simulink model "ChiefMaster_TTC580"  (R2022b)
settings: Solver=FixedStepAuto  StartTime=0.0  StopTime=10  FixedStep=0.01  RelTol=1e-3
values from neighbouring files (symbols this model uses):
  BattBox1_No = single(1)    [Parameters.m]
  BattBox2_No = single(2)    [Parameters.m]
  BattBox3_No = single(3)    [Parameters.m]
  CurrentLB = single(-3)    [Parameters.m]
  CurrentReductionConstant_Lvl0 = single(0.03)    [Parameters.m]
  CurrentReductionConstant_Lvl1 = single(0.05)    [Parameters.m]
  CurrentReductionConstant_Lvl2 = single(0.07)    [Parameters.m]
  CurrentReductionConstant_Lvl3 = single(0.1)    [Parameters.m]
  CurrentUB = single(3)    [Parameters.m]
  DCHV_Minus_In_Delay_ms = single(500)    [Parameters.m]
  FL_sHVC_CellBalanceVoltage_mV = single(3500)    [Parameters.m]
  FL_sInrushCurrent_dividebyzero = single(0.00001)    [Parameters.m]
  FL_u8HMI_BuzzerTimer = uint8(3)    [Parameters.m]
  IP_boActValue = true    [Parameters.m]
  IP_boDeactValue = false    [Parameters.m]
  IP_boInitValue = false    [Parameters.m]
  IP_s_LB = 18000    [Parameters.m]
  IP_s_UB = 22000    [Parameters.m]
  IP_sBatt1_ChargeCurrentMax_Factor = single(0.1)    [Parameters.m]
  IP_sBatt1_ChargeCurrentMax_LB = single(0)    [Parameters.m]
  IP_sBatt1_ChargeCurrentMax_Offset = single(0)    [Parameters.m]
  IP_sBatt1_ChargeCurrentMax_UB = single(6553.5)    [Parameters.m]
  IP_sBatt1_Current_Factor = single(0.1)    [Parameters.m]
  IP_sBatt1_Current_LB = single(-3276.8)    [Parameters.m]
  IP_sBatt1_Current_Offset = single(0)    [Parameters.m]
  IP_sBatt1_Current_UB = single(3276.8)    [Parameters.m]
  IP_sBatt1_DisChargeCurrentMax_Factor = single(0.1)    [Parameters.m]
  IP_sBatt1_DisChargeCurrentMax_LB = single(0)    [Parameters.m]
  IP_sBatt1_DisChargeCurrentMax_Offset = single(0)    [Parameters.m]
  IP_sBatt1_DisChargeCurrentMax_UB = single(6553.5)    [Parameters.m]
  IP_sBatt1_InsulationResistance_Factor = single(5)    [Parameters.m]
  IP_sBatt1_InsulationResistance_LB = single(0)    [Parameters.m]
  IP_sBatt1_InsulationResistance_Offset = single(0)    [Parameters.m]
  IP_sBatt1_InsulationResistance_UB = single(0)    [Parameters.m]
  IP_sBatt1_LiBa_IntResist_mOhm = single(25)    [Parameters.m]
  IP_sBatt1_SOC_Factor = single(1)    [Parameters.m]
  IP_sBatt1_SOC_LB = single(0)    [Parameters.m]
  IP_sBatt1_SOC_Offset = single(0)    [Parameters.m]
  IP_sBatt1_SOC_UB = single(100)    [Parameters.m]
  IP_sBatt1_SOH_Factor = single(1)    [Parameters.m]
  IP_sBatt1_SOH_LB = single(0)    [Parameters.m]
  IP_sBatt1_SOH_Offset = single(0)    [Parameters.m]
  IP_sBatt1_SOH_UB = single(100)    [Parameters.m]
  IP_sBatt1_Ubatt_Factor = single(0.1)    [Parameters.m]
  IP_sBatt1_Ubatt_LB = single(0)    [Parameters.m]
  IP_sBatt1_Ubatt_Offset = single(0)    [Parameters.m]
  IP_sBatt1_Ubatt_UB = single(6553.5)    [Parameters.m]
  IP_sBatt1_UserRi_Factor = single(1)    [Parameters.m]
  IP_sBatt1_UserRi_LB = single(0)    [Parameters.m]
  IP_sBatt1_UserRi_Offset = single(0)    [Parameters.m]
  IP_sBatt1_UserRi_UB = single(255)    [Parameters.m]
  IP_sBatt1_VoltageAtSensor_Factor = single(0.02)    [Parameters.m]
  IP_sBatt1_VoltageAtSensor_LB = single(0)    [Parameters.m]
  IP_sBatt1_VoltageAtSensor_Offset = single(0)    [Parameters.m]
  IP_sBatt1_VoltageAtSensor_UB = single(1310.7)    [Parameters.m]
  IP_sBatt2_LiBa_IntResist_mOhm = single(25)    [Parameters.m]
  IP_sBatt3_LiBa_IntResist_mOhm = single(25)    [Parameters.m]
  IP_sEM_LB = 2000    [Parameters.m]
  IP_sEM_UB = 8000    [Parameters.m]
  IP_sFB_LB = 5000    [Parameters.m]
  IP_sFB_UB = 10000    [Parameters.m]
  IP_sHVIL_LB = 12000    [Parameters.m]
  IP_sHVIL_UB = 15000    [Parameters.m]
  IP_sLoad_Voltage_Factor = single(1)    [Parameters.m]
  IP_sLoad_Voltage_LB = single(0)    [Parameters.m]
  IP_sLoad_Voltage_Offset = single(0)    [Parameters.m]
  IP_sLoad_Voltage_UB = single(65535)    [Parameters.m]
  IP_u8HVIL_Delay_ms = uint8(100)    [Parameters.m]
  IP_u8HW_IN_delay_ms = uint8(100)    [Parameters.m]
  IT_sInsulationSafeValue_kOhm = single(650)    [Parameters.m]
  IT_u8IMD_DelayTime_s = uint8(20)    [Parameters.m]
  MainHV_Minus_In_Delay = single(5)    [Parameters.m]
  MainHV_StatusDelay = single(5)    [Parameters.m]
  NotAvailable_uint16 = single(65535)    [Parameters.m]
  NotAvailable_uint8 = uint8(255)    [Parameters.m]
  OP_boHVIL_Supply = boolean(1)    [Parameters.m]
  SafeCurrentToCloseHV_A = single(5)    [Parameters.m]
  SafeVoltageToCloseHV_V = single(0.5)    [Parameters.m]
  UnexpectedBattChargingFcn_Available = boolean(1)    [Parameters.m]
  Voltage_NA_UB = uint16(65535)    [Parameters.m]
  VoltageSensorAvailableBB1 = boolean(0)    [Parameters.m]
  VoltageSensorAvailableBB2 = boolean(0)    [Parameters.m]
  VoltageSensorAvailableBB3 = boolean(0)    [Parameters.m]
libraries: simulink x184, Library_DataProcessing_v1_1 x167, Library_DataProcessing_v1 x142, libCM x28
(part 3 of 19)

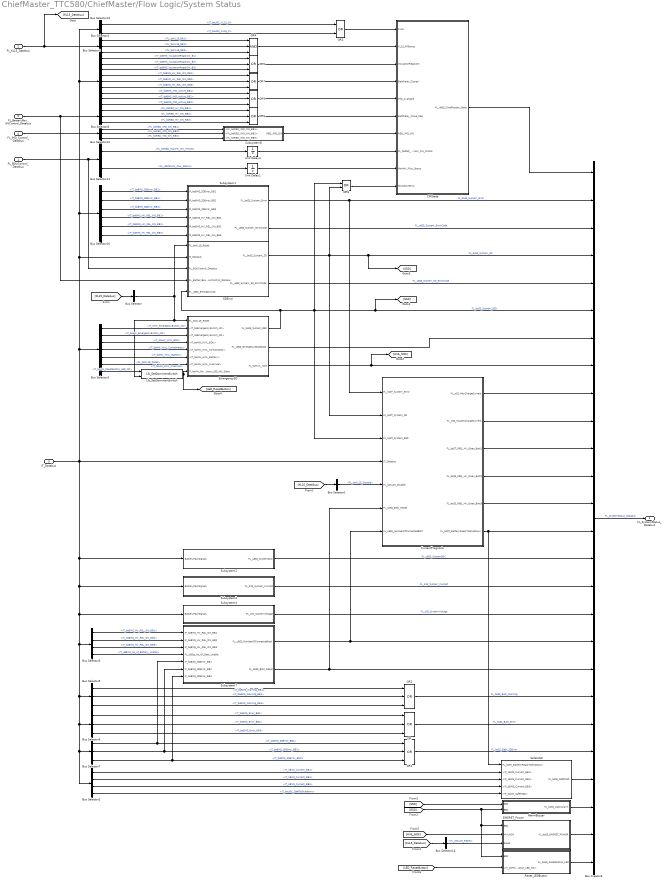
== system ChiefMaster_TTC580/ChiefMaster/Flow Logic/System Status ==
  FL_BDUControl_Databus : Inport
  FL_KL15_Databus : Inport  Port=2
  IT_Databus : Inport  Port=3
  FL_IMD_Control_Databus : Inport  Port=4
  FL_BatteryBox_HVControl_Databus : Inport  Port=5
  AlarmBuzzer : Subsystem
  Bus Creator6 : BusCreator  Inputs=26
  Bus Selector : BusSelector  OutputSignals=FL_boKL15_Reset
  Bus Selector1 : BusSelector  OutputSignals=FL_boKL15_Disable
  Bus Selector10 : BusSelector  OutputSignals=IT_BatterySignal_Databus.IT_boBMS_SDError_BB1,IT_BatterySignal_Databus.IT_boBMS_SDError_BB2,IT_BatterySignal_Databus.IT_boBMS_SDError_BB3,IT_BatterySignal_Databus.IT_boBMS_HV_REL_ON_BB1,IT_BatterySignal_Databus.IT_boBMS_HV_REL_ON_BB2,IT_BatterySignal_Databus.IT_boBMS_HV_REL_ON_BB3
  Bus Selector11 : BusSelector  OutputSignals=FL_boREQ_MainHV_ON_MINUS,FL_u8MainHV_Plus_Status
  Bus Selector12 : BusSelector  OutputSignals=FL_boREQ_IMD_ON_BB1,FL_boREQ_IMD_ON_BB2,FL_boREQ_IMD_ON_BB3
  Bus Selector13 : BusSelector  OutputSignals=IT_UDC_Databus.IT_boUDC_KL15_D,IT_UDC_Databus.IT_boUDC_KL15_C
  Bus Selector14 : BusSelector  OutputSignals=FL_boKL15_Reset
  Bus Selector2 : BusSelector  OutputSignals=IT_BatterySignal_Databus.IT_sBMS_Current_BB1,IT_BatterySignal_Databus.IT_sBMS_Current_BB2,IT_BatterySignal_Databus.IT_sBMS_Current_BB3,IT_UDC_Databus.IT_boUDC_SafeToShutdown
  Bus Selector3 : BusSelector  OutputSignals=IT_HW_Input_Databus.IT_sHW_EmergencyButton_NC,IT_HW_Input_Databus.IT_boHW_EmergencyButton_NO,IT_HW_Input_Databus.IT_boHW_HVIL_BDU,IT_HW_Input_Databus.IT_boHW_HVIL_Components,IT_HW_Input_Databus.IT_boHW_HVIL_Battery,IT_HW_Input_Databus.IT_boHW_HVIL_Overrule,IT_HW_Input_Databus.IT_boHW_ResetButton_LED_NO
  "Bus Selector3 " : BusSelector  OutputSignals=IT_BatterySignal_Databus.IT_boBMS_HV_REL_ON_BB1,IT_BatterySignal_Databus.IT_boBMS_HV_REL_ON_BB2,IT_BatterySignal_Databus.IT_boBMS_HV_REL_ON_BB3,IT_BatterySignal_Databus.IT_u8BMS_No_of_Battery_Usable
  Bus Selector4 : BusSelector  OutputSignals=FL_boKL15_BB1,FL_boKL15_BB2,FL_boKL15_BB3
  Bus Selector5 : BusSelector  OutputSignals=IT_BatterySignal_Databus.IT_boBMS_Warning_BB1,IT_BatterySignal_Databus.IT_boBMS_Warning_BB2,IT_BatterySignal_Databus.IT_boBMS_Warning_BB3
  Bus Selector6 : BusSelector  OutputSignals=IT_BatterySignal_Databus.IT_boBMS_Error_BB1,IT_BatterySignal_Databus.IT_boBMS_Error_BB2,IT_BatterySignal_Databus.IT_boBMS_Error_BB3
  Bus Selector7 : BusSelector  OutputSignals=IT_BatterySignal_Databus.IT_boBMS_SDError_BB1,IT_BatterySignal_Databus.IT_boBMS_SDError_BB2,IT_BatterySignal_Databus.IT_boBMS_SDError_BB3
  Bus Selector8 : BusSelector  OutputSignals=FL_boREQ_HV_ON_BB1,FL_boREQ_HV_ON_BB2,FL_boREQ_HV_ON_BB3
  Bus Selector9 : BusSelector  OutputSignals=IT_BatterySignal_Databus.IT_boBMS_InsulationReadyOK_B1,IT_BatterySignal_Databus.IT_boBMS_InsulationReadyOK_B2,IT_BatterySignal_Databus.IT_boBMS_InsulationReadyOK_B3,IT_BatterySignal_Databus.IT_boBMS_HV_REL_ON_BB1,IT_BatterySignal_Databus.IT_boBMS_HV_REL_ON_BB2,IT_BatterySignal_Databus.IT_boBMS_HV_REL_ON_BB3,IT_BatterySignal_Databus.IT_boBMS_IMD_Active_BB1,IT_BatterySignal_Databus.IT_boBMS_IMD_Active_BB2,IT_BatterySignal_Databus.IT_boBMS_IMD_Active_BB3
  CMState : Subsystem  TreatAsAtomicUnit=on
      settings: RTWFcnNameOpts=Use subsystem name  RTWFileNameOpts=Use subsystem name
  CurrentPrognosis : Subsystem
  EMSRET_Power : Subsystem  TreatAsAtomicUnit=on
      settings: RTWFcnNameOpts=Use subsystem name  RTWFileNameOpts=Use subsystem name
  EmergencySD : Subsystem  TreatAsAtomicUnit=on
      settings: RTWFcnNameOpts=Use subsystem name  RTWFileNameOpts=Use subsystem name
  Lib_SetDominantSwitch : Library_DataProcessing_v1_1/Lib_SetDominantSwitch  SystemSampleTime=-1  VariantActivationTime=update diagram  Latency=0  AutoFrameSizeCalculation=off
  OR{,1..2,5..7,9} (7 alike) : Logic  Operator=OR  Inputs=3  AllPortsSameDT=off  OutDataTypeStr=boolean
  OR3 : Logic  Operator=OR  AllPortsSameDT=off  OutDataTypeStr=boolean
  OR4 : Logic  Inputs=3  AllPortsSameDT=off  OutDataTypeStr=boolean
  OR8 : Logic  Operator=OR  AllPortsSameDT=off  OutDataTypeStr=boolean
  Reset_LEDButton : Subsystem
  SDError : Subsystem  TreatAsAtomicUnit=on
      settings: RTWFcnNameOpts=Use subsystem name  RTWFileNameOpts=Use subsystem name
  SafetoSD : Subsystem
  Subsystem1 : Subsystem
  Subsystem2 : Subsystem
  Subsystem3 : Subsystem
  Subsystem4 : Subsystem
  Subsystem7 : Subsystem
  Subsystem8 : Subsystem
  Unit Delay1 : UnitDelay  SampleTime=-1  HasFrameUpgradeWarning=on
  Unit Delay4 : UnitDelay  SampleTime=-1  HasFrameUpgradeWarning=on
  FL_SystemStatus_Databus : Outport
  wires:
  "Bus Selector3 "/4 -> Subsystem7/4(FL_u8Sig_No_Of_Batt_Usable)  "<IT_u8BMS_No_of_Battery_Usable>"
  Subsystem1/2(FL_u8SS_System_ErrorCode) -> Bus Creator6/3  "FL_u8SS_System_ErrorCode"
  Bus Selector10/4 -> Subsystem1/4(IP_boBMS_HV_REL_ON_BB1)  "<IT_boBMS_HV_REL_ON_BB1>"
  Subsystem7/1(FL_u8SS_NumberOfConnectedBatt) -> CurrentPrognosis/7(FL_u8SS_NumberOfConnectedBatt), Bus Creator6/18
  Bus Selector10/6 -> Subsystem1/6(IP_boBMS_HV_REL_ON_BB3)  "<IT_boBMS_HV_REL_ON_BB3>"
  Bus Selector5/1 -> OR2/1  "<IT_boBMS_Warning_BB1>"
  Subsystem1/1(FL_boSS_System_Error) -> CurrentPrognosis/1(FL_boST_System_Error), Bus Creator6/2  "FL_boSS_System_Error"
  "Bus Selector3 "/2 -> Subsystem7/2(IP_boBMS_HV_REL_ON_BB2)  "<IT_boBMS_HV_REL_ON_BB2>"
  SDError/2(FL_u8SS_System_SD_ErrorCode) -> Bus Creator6/5  "FL_u8SS_System_SD_ErrorCode"
  "Bus Selector3 "/1 -> Subsystem7/1(IP_boBMS_HV_REL_ON_BB1)  "<IT_boBMS_HV_REL_ON_BB1>"
  Bus Selector10/5 -> Subsystem1/5(IP_boBMS_HV_REL_ON_BB2)  "<IT_boBMS_HV_REL_ON_BB2>"
  Bus Selector10/1 -> Subsystem1/1(IP_boBMS_SDError_BB1)  "<IT_boBMS_SDError_BB1>"
  Bus Selector7/1 -> OR1/1, Subsystem7/5(IP_boBMS_SDError_BB1)  "<IT_boBMS_SDError_BB1>"
  "Bus Selector3 "/3 -> Subsystem7/3(IP_boBMS_HV_REL_ON_BB3)  "<IT_boBMS_HV_REL_ON_BB3>"
  Bus Selector5/2 -> OR2/2  "<IT_boBMS_Warning_BB2>"
  Bus Selector6/3 -> OR/3  "<IT_boBMS_Error_BB3>"
  Bus Selector7/3 -> Subsystem7/7(IP_boBMS_SDError_BB3), OR1/3  "<IT_boBMS_SDError_BB3>"
  Subsystem7/2(FL_boSS_BDU_Reset) -> CurrentPrognosis/6(FL_boSS_BDU_Reset), Bus Creator6/19
  Bus Selector6/2 -> OR/2  "<IT_boBMS_Error_BB2>"
  Bus Selector10/3 -> Subsystem1/3(IP_boBMS_SDError_BB3)  "<IT_boBMS_SDError_BB3>"
  OR2/1 -> Bus Creator6/20  "FL_boSS_Batt_Warning"
  OR1/1 -> Bus Creator6/22  "FL_boSS_Batt_SDError"
  Bus Selector10/2 -> Subsystem1/2(IP_boBMS_SDError_BB2)  "<IT_boBMS_SDError_BB2>"
  Bus Selector5/3 -> OR2/3  "<IT_boBMS_Warning_BB3>"
  Bus Selector6/1 -> OR/1  "<IT_boBMS_Error_BB1>"
  OR/1 -> Bus Creator6/21  "FL_boSS_Batt_Error"
  Subsystem4/1(FL_sST_SystemVoltage) -> Bus Creator6/17  "FL_sSS_SystemVoltage"
  Bus Creator6/1 -> FL_SystemStatus_Databus/1  "FL_SystemStatus_Databus"
  Bus Selector/1 -> Lib_SetDominantSwitch/2, EmergencySD/1(FL_boKL15_Reset), SDError/1(FL_boKL15_Reset)  "<FL_boKL15_Reset>"
  FL_BatteryBox_HVControl_Databus/1 -> SDError/4(FL_BatteryBox_HVControl_Databus), Bus Selector8/1
  Subsystem3/1(FL_sSS_System_Current) -> Bus Creator6/16  "FL_sSS_System_Current"
  Subsystem2/1(FL_u8SS_SystemSOC) -> Bus Creator6/15  "FL_u8SS_SystemSOC"
  CurrentPrognosis/1(FL_sSS_MaxChargeCurrent) -> Bus Creator6/9
  EmergencySD/1(FL_boSS_System_ESD) -> SDError/5(FL_u8SS_EmergencySD), CurrentPrognosis/3(FL_boST_System_ESD), OR8/1, [ESD], Bus Creator6/6  "FL_boSS_System_ESD"
  Bus Selector3/1 -> EmergencySD/2(<IT_boEmergencySwitch_NC>)  "<IT_sHW_EmergencyButton_NC>"
  SDError/1(FL_boSS_System_SD) -> OR8/2, [SSD], Bus Creator6/4, CurrentPrognosis/2(FL_boST_System_SD)  "FL_boSS_System_SD"
  Bus Selector7/2 -> Subsystem7/6(IP_boBMS_SDError_BB2), OR1/2  "<IT_boBMS_SDError_BB2>"
  CurrentPrognosis/2(FL_sSS_MaxDisChargeCurrent) -> Bus Creator6/10
  OR9/1 -> CMState/5(IMD_Available)
  Bus Selector9/9 -> OR9/3  "<IT_boBMS_IMD_Active_BB3>"
  Bus Selector9/8 -> OR9/2  "<IT_boBMS_IMD_Active_BB2>"
  Bus Selector9/7 -> OR9/1  "<IT_boBMS_IMD_Active_BB1>"
  Subsystem8/1(REQ_IMD_ON) -> CMState/7(REQ_IMD_ON)
  OR6/1 -> CMState/6(BattRelay_Close_Req)
  OR7/1 -> CMState/4(BattRelay_Closed)
  OR5/1 -> CMState/3(InsulationReadyOK)
  Unit Delay1/1 -> CMState/9(MainHV_Plus_Status)
  Bus Selector12/3 -> Subsystem8/3(<FL_boREQ_IMD_ON_BB3>)  "<FL_boREQ_IMD_ON_BB3>"
  Bus Selector12/2 -> Subsystem8/2(<FL_boREQ_IMD_ON_BB2>)  "<FL_boREQ_IMD_ON_BB2>"
  Bus Selector12/1 -> Subsystem8/1(<FL_boREQ_IMD_ON_BB1>)  "<FL_boREQ_IMD_ON_BB1>"
  OR4/1 -> CMState/2(KL15_AllBoxes)
  Unit Delay4/1 -> CMState/8(FL_boREQ_MainHV_ON_MINUS)
  OR8/1 -> CMState/10(ShutdownError)
  Bus Selector9/6 -> OR7/3  "<IT_boBMS_HV_REL_ON_BB3>"
  Bus Selector9/5 -> OR7/2  "<IT_boBMS_HV_REL_ON_BB2>"
  Bus Selector9/4 -> OR7/1  "<IT_boBMS_HV_REL_ON_BB1>"
  Bus Selector11/2 -> Unit Delay1/1  "<FL_u8MainHV_Plus_Status>"
  Bus Selector11/1 -> Unit Delay4/1  "<FL_boREQ_MainHV_ON_MINUS>"
  FL_BDUControl_Databus/1 -> Bus Selector11/1, SDError/3(FL_BDUControl_Databus)
  Bus Selector8/3 -> OR6/3  "<FL_boREQ_HV_ON_BB3>"
  Bus Selector8/2 -> OR6/2  "<FL_boREQ_HV_ON_BB2>"
  Bus Selector8/1 -> OR6/1  "<FL_boREQ_HV_ON_BB1>"
  Bus Selector9/3 -> OR5/3  "<IT_boBMS_InsulationReadyOK_B3>"
  Bus Selector9/2 -> OR5/2  "<IT_boBMS_InsulationReadyOK_B2>"
  Bus Selector9/1 -> OR5/1  "<IT_boBMS_InsulationReadyOK_B1>"
  IT_Databus/1 -> SDError/2(IT_Databus), Bus Selector13/1, Bus Selector9/1, Bus Selector10/1, Bus Selector3/1, Subsystem4/1(BatteryPackSignals), Bus Selector2/1, Bus Selector7/1, Bus Selector6/1, Bus Selector5/1, "Bus Selector3 "/1, Subsystem3/1(BatteryPackSignals), Subsystem2/1(BatteryPackSignals), CurrentPrognosis/4(IT_Databus)
  Bus Selector4/3 -> OR4/3  "<FL_boKL15_BB3>"
  Bus Selector4/2 -> OR4/2  "<FL_boKL15_BB2>"
  Bus Selector4/1 -> OR4/1  "<FL_boKL15_BB1>"
  FL_KL15_Databus/1 -> [KL15_Databus], Bus Selector4/1
  FL_IMD_Control_Databus/1 -> Bus Selector12/1
  CMState/1(FL_u8SS_ChiefMaster_State) -> Bus Creator6/1
  Bus Selector13/1 -> OR3/1  "<IT_boUDC_KL15_D>"
  Bus Selector3/2 -> EmergencySD/3(<IT_boEmergencySwitch_NO>)  "<IT_boHW_EmergencyButton_NO>"
  EmergencySD/2(FL_u8SS_EmergencyStopState) -> Bus Creator6/7
  [KL15_Databus] -> Bus Selector/1
  Bus Selector1/1 -> CurrentPrognosis/5(FL_boKL15_Disable)  "<FL_boKL15_Disable>"
  [KL15_Databus] -> Bus Selector1/1
  CurrentPrognosis/3(FL_boST_REQ_HV_Open_Batt1) -> Bus Creator6/11
  CurrentPrognosis/4(FL_boSS_REQ_HV_Open_Batt2) -> Bus Creator6/12
  CurrentPrognosis/5(FL_boSS_REQ_HV_Open_Batt3) -> Bus Creator6/13
  CurrentPrognosis/6(FL_boST_BatteryReadyToShutDown) -> Bus Creator6/14, SafetoSD/1(FL_boST_BatteryReadyToShutDown)
  SafetoSD/1(FL_boSS_SafeToSD) -> Bus Creator6/23
  Bus Selector2/1 -> SafetoSD/2(<IP_sBMS_Current_BB1>)  "<IT_sBMS_Current_BB1>"
  Bus Selector2/2 -> SafetoSD/3(<IP_sBMS_Current_BB2>)  "<IT_sBMS_Current_BB2>"
  Bus Selector2/3 -> SafetoSD/4(<IP_sBMS_Current_BB3>)  "<IT_sBMS_Current_BB3>"
  Bus Selector2/4 -> SafetoSD/5(<IP_boCM_SafeToSD>)  "<IT_boUDC_SafeToShutdown>"
  Bus Selector3/3 -> EmergencySD/4(<IT_boHW_HVIL_BDU>)  "<IT_boHW_HVIL_BDU>"
  Bus Selector3/4 -> EmergencySD/5(<IT_boHW_HVIL_Components>)  "<IT_boHW_HVIL_Components>"
  Bus Selector3/5 -> EmergencySD/6(<IT_boHW_HVIL_Battery>)  "<IT_boHW_HVIL_Battery>"
  Bus Selector3/6 -> EmergencySD/7(<IT_boHW_HVIL_Overrule>)  "<IT_boHW_HVIL_Overrule>"
  EmergencySD/3(FL_boHVIL_NOK) -> [HVIL_NOK], Bus Creator6/8
  [ESD] -> Reset_LEDButton/1(ESD), EMSRET_Power/1(ESD), AlarmBuzzer/2(ESD)
  EMSRET_Power/1(FL_boSS_EMSRET_POWER) -> Bus Creator6/25
  AlarmBuzzer/1(FL_boSS_CabinAlarm) -> Bus Creator6/24
  [HVIL_NOK] -> EMSRET_Power/2(HVILNOK)
  [SSD] -> AlarmBuzzer/1(SSD)
  Bus Selector14/1 -> EMSRET_Power/3(Reset)  "<FL_boKL15_Reset>"
  [KL15_Databus] -> Bus Selector14/1
  Bus Selector13/2 -> OR3/2  "<IT_boUDC_KL15_C>"
  OR3/1 -> CMState/1(KL15)
  Bus Selector3/7 -> Lib_SetDominantSwitch/1  "<IT_boHW_ResetButton_LED_NO>"
  Reset_LEDButton/1(FL_boSS_ResetButton_LED) -> Bus Creator6/26
  Lib_SetDominantSwitch/1 -> EmergencySD/8(IT_boHW_ResetButton_LED_NO_State), [LED_ResetButton]
  [LED_ResetButton] -> Reset_LEDButton/2(<IT_boHW_ResetButton_LED_NO>)

== system ChiefMaster_TTC580/ChiefMaster/Input Processing/Actia ==
  C_Actia_Batt1_MyStatus : Inport  OutDataTypeStr=uint8
  C_Actia_Batt1_MyStatus_Timeout : Inport  Port=2  OutDataTypeStr=boolean
  C_Actia_Batt1_Error : Inport  Port=3  OutDataTypeStr=uint8
  C_Actia_Batt1_Error_Timeout : Inport  Port=4  OutDataTypeStr=boolean
  C_Actia_Batt1_ADS_8 : Inport  Port=5  OutDataTypeStr=uint8
  C_Actia_Batt1_ADS_8_Timeout : Inport  Port=6  OutDataTypeStr=boolean
  C_Actia_Batt1_ADS_0 : Inport  Port=7
  C_Actia_Batt1_ADS_0_Timeout : Inport  Port=8
  C_Actia_Batt1_ADS_1 : Inport  Port=9  OutDataTypeStr=uint8
  C_Actia_Batt1_ADS_1_Timeout : Inport  Port=10  OutDataTypeStr=boolean
  C_Actia_Batt1_ADS_3 : Inport  Port=11  OutDataTypeStr=uint8
  C_Actia_Batt1_ADS_3_Timeout : Inport  Port=12  OutDataTypeStr=boolean
  C_Actia_Batt2_MyStatus : Inport  Port=13  OutDataTypeStr=uint8
  C_Actia_Batt2_MyStatus_Timeout : Inport  Port=14  OutDataTypeStr=boolean
  C_Actia_Batt2_Error : Inport  Port=15  OutDataTypeStr=uint8
  C_Actia_Batt2_Error_Timeout : Inport  Port=16  OutDataTypeStr=boolean
  C_Actia_Batt2_ADS_8 : Inport  Port=17  OutDataTypeStr=uint8
  C_Actia_Batt2_ADS_8_Timeout : Inport  Port=18  OutDataTypeStr=boolean
  C_Actia_Batt2_ADS_0 : Inport  Port=19
  C_Actia_Batt2_ADS_0_Timeout : Inport  Port=20
  C_Actia_Batt2_ADS_1 : Inport  Port=21  OutDataTypeStr=uint8
  C_Actia_Batt2_ADS_1_Timeout : Inport  Port=22  OutDataTypeStr=boolean
  C_Actia_Batt2_ADS_3 : Inport  Port=23  OutDataTypeStr=uint8
  C_Actia_Batt2_ADS_3_Timeout : Inport  Port=24  OutDataTypeStr=boolean
  C_Actia_Batt3_MyStatus : Inport  Port=25  OutDataTypeStr=uint8
  C_Actia_Batt3_MyStatus_Timeout : Inport  Port=26  OutDataTypeStr=boolean
  C_Actia_Batt3_Error : Inport  Port=27  OutDataTypeStr=uint8
  C_Actia_Batt3_Error_Timeout : Inport  Port=28  OutDataTypeStr=boolean
  C_Actia_Batt3_ADS_8 : Inport  Port=29  OutDataTypeStr=uint8
  C_Actia_Batt3_ADS_8_Timeout : Inport  Port=30  OutDataTypeStr=boolean
  C_Actia_Batt3_ADS_0 : Inport  Port=31
  C_Actia_Batt3_ADS_0_Timeout : Inport  Port=32
  C_Actia_Batt3_ADS_1 : Inport  Port=33  OutDataTypeStr=uint8
  C_Actia_Batt3_ADS_1_Timeout : Inport  Port=34  OutDataTypeStr=boolean
  C_Actia_Batt3_ADS_3 : Inport  Port=35  OutDataTypeStr=uint8
  C_Actia_Batt3_ADS_3_Timeout : Inport  Port=36  OutDataTypeStr=boolean
  Batt Box 1 : Subsystem
  Batt Box 2 : Subsystem
  Batt Box 3 : Subsystem
  Bus Creator : BusCreator  Inputs=3
  Actia_BattBox_dataBus : Outport
  wires:
  C_Actia_Batt3_ADS_3_Timeout/1 -> Batt Box 3/12(C_Actia_Batt3_ADS_3_Timeout)
  C_Actia_Batt1_ADS_0/1 -> Batt Box 1/7(C_Actia_Batt1_ADS_0)
  C_Actia_Batt1_ADS_0_Timeout/1 -> Batt Box 1/8(C_Actia_Batt1_ADS_0_Timeout)
  C_Actia_Batt1_MyStatus/1 -> Batt Box 1/1(C_Actia_Batt1_MyStatus)
  C_Actia_Batt1_MyStatus_Timeout/1 -> Batt Box 1/2(C_Actia_Batt1_MyStatus_Timeout)
  C_Actia_Batt1_Error/1 -> Batt Box 1/3(C_Actia_Batt1_Error)
  C_Actia_Batt1_Error_Timeout/1 -> Batt Box 1/4(C_Actia_Batt1_Error_Timeout)
  C_Actia_Batt1_ADS_8/1 -> Batt Box 1/5(C_Actia_Batt1_ADS_8)
  C_Actia_Batt1_ADS_8_Timeout/1 -> Batt Box 1/6(C_Actia_Batt1_ADS_8_Timeout)
  C_Actia_Batt1_ADS_1/1 -> Batt Box 1/9(C_Actia_Batt1_ADS_1)
  C_Actia_Batt1_ADS_3/1 -> Batt Box 1/11(C_Actia_Batt1_ADS_3)
  C_Actia_Batt1_ADS_1_Timeout/1 -> Batt Box 1/10(C_Actia_Batt1_ADS_1_Timeout)
  C_Actia_Batt2_MyStatus/1 -> Batt Box 2/1(C_Actia_Batt2_MyStatus)
  C_Actia_Batt1_ADS_3_Timeout/1 -> Batt Box 1/12(C_Actia_Batt1_ADS_3_Timeout)
  Bus Creator/1 -> Actia_BattBox_dataBus/1  "IP_Actia_BatBox_DataBus"
  C_Actia_Batt2_Error/1 -> Batt Box 2/3(C_Actia_Batt2_Error)
  C_Actia_Batt2_MyStatus_Timeout/1 -> Batt Box 2/2(C_Actia_Batt2_MyStatus_Timeout)
  C_Actia_Batt2_ADS_8/1 -> Batt Box 2/5(C_Actia_Batt2_ADS_8)
  C_Actia_Batt2_Error_Timeout/1 -> Batt Box 2/4(C_Actia_Batt2_Error_Timeout)
  C_Actia_Batt2_ADS_8_Timeout/1 -> Batt Box 2/6(C_Actia_Batt2_ADS_8_Timeout)
  C_Actia_Batt2_ADS_0/1 -> Batt Box 2/7(C_Actia_Batt2_ADS_0)
  C_Actia_Batt2_ADS_3_Timeout/1 -> Batt Box 2/12(C_Actia_Batt2_ADS_3_Timeout)
  C_Actia_Batt2_ADS_3/1 -> Batt Box 2/11(C_Actia_Batt2_ADS_3)
  C_Actia_Batt2_ADS_0_Timeout/1 -> Batt Box 2/8(C_Actia_Batt2_ADS_0_Timeout)
  C_Actia_Batt2_ADS_1_Timeout/1 -> Batt Box 2/10(C_Actia_Batt2_ADS_1_Timeout)
  C_Actia_Batt2_ADS_1/1 -> Batt Box 2/9(C_Actia_Batt2_ADS_1)
  C_Actia_Batt3_MyStatus/1 -> Batt Box 3/1(C_Actia_Batt3_MyStatus)
  C_Actia_Batt3_Error/1 -> Batt Box 3/3(C_Actia_Batt3_Error)
  C_Actia_Batt3_MyStatus_Timeout/1 -> Batt Box 3/2(C_Actia_Batt3_MyStatus_Timeout)
  C_Actia_Batt3_ADS_8/1 -> Batt Box 3/5(C_Actia_Batt3_ADS_8)
  C_Actia_Batt3_Error_Timeout/1 -> Batt Box 3/4(C_Actia_Batt3_Error_Timeout)
  C_Actia_Batt3_ADS_8_Timeout/1 -> Batt Box 3/6(C_Actia_Batt3_ADS_8_Timeout)
  C_Actia_Batt3_ADS_3/1 -> Batt Box 3/11(C_Actia_Batt3_ADS_3)
  C_Actia_Batt3_ADS_1/1 -> Batt Box 3/9(C_Actia_Batt3_ADS_1)
  C_Actia_Batt3_ADS_1_Timeout/1 -> Batt Box 3/10(C_Actia_Batt3_ADS_1_Timeout)
  Batt Box 1/1(IP_Actia_Batt1_Databus) -> Bus Creator/1
  Batt Box 2/1(IP_Actia_Batt2_Databus) -> Bus Creator/2
  Batt Box 3/1(IP_Actia_Batt3_Databus) -> Bus Creator/3
  C_Actia_Batt3_ADS_0_Timeout/1 -> Batt Box 3/8(C_Actia_Batt3_ADS_0_Timeout)
  C_Actia_Batt3_ADS_0/1 -> Batt Box 3/7(C_Actia_Batt3_ADS_0)

== system ChiefMaster_TTC580/ChiefMaster/Input Processing/HW Inputs ==
  AI_KL15 : Inport
  AI_HVIL_BDU : Inport  Port=2  OutDataTypeStr=single
  AI_HVIL_Component : Inport  Port=3  OutDataTypeStr=single
  AI_HVIL_Battery : Inport  Port=4  OutDataTypeStr=single
  DI_HVIL_Overrule : Inport  Port=5  OutDataTypeStr=boolean
  AI_MainHV_Plus_FB : Inport  Port=6
  AI_MainHV_Minus_FB : Inport  Port=7
  AI_EmergencyButton_NC : Inport  Port=8  OutDataTypeStr=single
  AI_EmergencyButton_NO : Inport  Port=9
  DI_ResetButton_LED_NO : Inport  Port=10
  DI_Proximity_BB1 : Inport  Port=11
  DI_Proximity_BB2 : Inport  Port=12
  DI_Proximity_BB3 : Inport  Port=13
  AI_DCHV_Plus_FB : Inport  Port=14
  AI_DCHV_Minus_FB : Inport  Port=15
  DI_IMD_FB_BB1 : Inport  Port=16
  DI_IMD_FB_BB2 : Inport  Port=17
  DI_IMD_FB_BB3 : Inport  Port=18
  Bus Creator : BusCreator  Inputs=18
  EmergencyButtonNC : Subsystem  TreatAsAtomicUnit=on
  EmergencyButtonNO : Subsystem  TreatAsAtomicUnit=on
  HVIL : Subsystem  TreatAsAtomicUnit=on
  HVIL1 : Subsystem  TreatAsAtomicUnit=on
  HVIL2 : Subsystem  TreatAsAtomicUnit=on
  Ignition : Subsystem  TreatAsAtomicUnit=on
  Minus_FB : Subsystem  TreatAsAtomicUnit=on
  Minuus_FB1 : Subsystem  TreatAsAtomicUnit=on
  Plus_FB : Subsystem  TreatAsAtomicUnit=on
  Plus_FB1 : Subsystem  TreatAsAtomicUnit=on
  Subsystem : Subsystem
  Subsystem1 : Subsystem
  Subsystem2 : Subsystem
  IP_HW_Input_DataBus : Outport
  wires:
  Subsystem2/1(Out) -> Bus Creator/13  "IP_boHW_Proximity_BB3"
  AI_KL15/1 -> Ignition/1("AI_KL15 ")
  AI_MainHV_Plus_FB/1 -> Plus_FB/1(AI_MainHV_Plus_FB)
  AI_HVIL_BDU/1 -> HVIL/1(IP_sHW_HVIL_BDU)
  HVIL1/1(IP_boHW_HVIL_Components) -> Bus Creator/3  "IP_boHW_HVIL_Components"
  AI_MainHV_Minus_FB/1 -> Minus_FB/1(AI_MainHV_Minus_FB)
  AI_EmergencyButton_NC/1 -> EmergencyButtonNC/1("EmergencyButton_NC ")
  HVIL2/1(IP_boHW_HVIL_Battery) -> Bus Creator/4  "IP_boHW_HVIL_Battery"
  AI_EmergencyButton_NO/1 -> EmergencyButtonNO/1("EmergencyButton_NO ")
  DI_ResetButton_LED_NO/1 -> Bus Creator/10  "IP_boHW_ResetButton_LED_NO"
  Subsystem/1(Out) -> Bus Creator/11  "IP_boHW_Proximity_BB1"
  Subsystem1/1(Out) -> Bus Creator/12  "IP_boHW_Proximity_BB2"
  AI_DCHV_Minus_FB/1 -> Minuus_FB1/1(AI_DCHV_Minus_FB)
  AI_DCHV_Plus_FB/1 -> Plus_FB1/1(AI_DCHV_Plus_FB)
  Bus Creator/1 -> IP_HW_Input_DataBus/1  "IP_HW_Input_DataBus"
  Ignition/1(IP_boHW_KL15) -> Bus Creator/1  "IP_boHW_KL15"
  EmergencyButtonNO/1(IP_boHW_EmergencyButton_NO) -> Bus Creator/9  "IP_boHW_EmergencyButton_NO"
  EmergencyButtonNC/1(IP_boHW_EmergencyButton_NC) -> Bus Creator/8  "IP_boHW_EmergencyButton_NC"
  DI_HVIL_Overrule/1 -> Bus Creator/5  "IP_boHW_HVIL_Overrule"
  HVIL/1(IP_boHW_HVIL_BDU) -> Bus Creator/2  "IP_boHW_HVIL_BDU"
  AI_HVIL_Component/1 -> HVIL1/1(IP_sHW_HVIL_BDU)
  AI_HVIL_Battery/1 -> HVIL2/1(IP_sHW_HVIL_BDU)
  DI_IMD_FB_BB1/1 -> Bus Creator/16  "IP_boHW_IMD_FB_BB1"
  DI_IMD_FB_BB2/1 -> Bus Creator/17  "IP_boHW_IMD_FB_BB2"
  DI_IMD_FB_BB3/1 -> Bus Creator/18  "IP_boHW_IMD_FB_BB3"
  Plus_FB/1(IP_boHW_MainHV_Plus_FB) -> Bus Creator/6  "IP_boHW_MainHV_Plus_FB"
  Minus_FB/1(IP_boHW_MainHV_Minus_FB) -> Bus Creator/7  "IP_boHW_MainHV_Minus_FB"
  Plus_FB1/1(IP_boHW_DCHV_Plus_FB) -> Bus Creator/14  "IP_boHW_DCHV_Plus_FB"
  Minuus_FB1/1(IP_boHW_DCHV_Minus_FB) -> Bus Creator/15  "IP_boHW_DCHV_Minus_FB"
  DI_Proximity_BB1/1 -> Subsystem/1(In)  "IP_boHW_Proximity_BB1"
  DI_Proximity_BB2/1 -> Subsystem1/1(DI_Proximity_BB2)  "IP_boHW_Proximity_BB2"
  DI_Proximity_BB3/1 -> Subsystem2/1(DI_Proximity_BB2)  "IP_boHW_Proximity_BB3"

== system ChiefMaster_TTC580/ChiefMaster/Input Processing/LiBa ==
  C_LB_Batt1_CellVoltage01_Msg : Inport
  C_LB_Batt1_CellVoltage01_Timeout : Inport  Port=2
  C_LB_Batt1_CellVoltage02_Msg : Inport  Port=3
  C_LB_Batt1_CellVoltage02_Timeout : Inport  Port=4
  C_LB_Batt1_CellTemperature_Msg : Inport  Port=5
  C_LB_Batt1_CellTemperature_Timeout : Inport  Port=6
  C_LB_Batt1_InsulationMonitor_Msg : Inport  Port=7
  C_LB_Batt1_InsulationMonitor_Timeout : Inport  Port=8
  C_LB_Batt1_Status01_Msg : Inport  Port=9
  C_LB_Batt1_Status01_Timeout : Inport  Port=10
  C_LB_Batt1_Status02_Msg : Inport  Port=11
  C_LB_Batt1_Status02_Timeout : Inport  Port=12
  C_LB_Batt1_Status03_Msg : Inport  Port=13
  C_LB_Batt1_Status03_Timeout : Inport  Port=14
  C_LB_Batt2_CellVoltage01_Msg : Inport  Port=15
  C_LB_Batt2_CellVoltage01_Timeout : Inport  Port=16
  C_LB_Batt2_CellVoltage02_Msg : Inport  Port=17
  C_LB_Batt2_CellVoltage02_Timeout : Inport  Port=18
  C_LB_Batt2_CellTemperature_Msg : Inport  Port=19
  C_LB_Batt2_CellTemperature_Timeout : Inport  Port=20
  C_LB_Batt2_InsulationMonitor_Msg : Inport  Port=21
  C_LB_Batt2_InsulationMonitor_Timeout : Inport  Port=22
  C_LB_Batt2_Status01_Msg : Inport  Port=23
  C_LB_Batt2_Status01_Timeout : Inport  Port=24
  C_LB_Batt2_Status02_Msg : Inport  Port=25
  C_LB_Batt2_Status02_Timeout : Inport  Port=26
  C_LB_Batt2_Status03_Msg : Inport  Port=27
  C_LB_Batt2_Status03_Timeout : Inport  Port=28
  C_LB_Batt3_CellVoltage01_Msg : Inport  Port=29
  C_LB_Batt3_CellVoltage01_Timeout : Inport  Port=30
  C_LB_Batt3_CellVoltage02_Msg : Inport  Port=31
  C_LB_Batt3_CellVoltage02_Timeout : Inport  Port=32
  C_LB_Batt3_CellTemperature_Msg : Inport  Port=33
  C_LB_Batt3_CellTemperature_Timeout : Inport  Port=34
  C_LB_Batt3_InsulationMonitor_Msg : Inport  Port=35
  C_LB_Batt3_InsulationMonitor_Timeout : Inport  Port=36
  C_LB_Batt3_Status01_Msg : Inport  Port=37
  C_LB_Batt3_Status01_Timeout : Inport  Port=38
  C_LB_Batt3_Status02_Msg : Inport  Port=39
  C_LB_Batt3_Status02_Timeout : Inport  Port=40
  C_LB_Batt3_Status03_Msg : Inport  Port=41
  C_LB_Batt3_Status03_Timeout : Inport  Port=42
  Bus Creator : BusCreator  Inputs=3
  LiBa_Box1 : Subsystem
  LiBa_Box2 : Subsystem
  LiBa_Box3 : Subsystem
  IP_LB_BattBox_DataBus : Outport
  wires:
  C_LB_Batt3_Status02_Timeout/1 -> LiBa_Box3/12(C_LB_Batt3_Status02_Timeout)
  C_LB_Batt3_CellVoltage01_Msg/1 -> LiBa_Box3/1(C_LB_Batt3_CellVoltage01_Msg)
  C_LB_Batt1_CellVoltage01_Timeout/1 -> LiBa_Box1/2(C_LB_Batt1_CellVoltage01_Timeout)
  C_LB_Batt2_CellVoltage01_Timeout/1 -> LiBa_Box2/2(C_LB_Batt2_CellVoltage01_Timeout)
  C_LB_Batt2_Status02_Timeout/1 -> LiBa_Box2/12(C_LB_Batt2_Status02_Timeout)
  C_LB_Batt2_CellVoltage02_Timeout/1 -> LiBa_Box2/4(C_LB_Batt2_CellVoltage02_Timeout)
  C_LB_Batt3_InsulationMonitor_Timeout/1 -> LiBa_Box3/8(C_LB_Batt3_InsulationMonitor_Timeout)
  C_LB_Batt2_Status03_Timeout/1 -> LiBa_Box2/14(C_LB_Batt2_Status03_Timeout)
  C_LB_Batt1_InsulationMonitor_Timeout/1 -> LiBa_Box1/8(C_LB_Batt1_InsulationMonitor_Timeout)
  C_LB_Batt2_CellVoltage02_Msg/1 -> LiBa_Box2/3(C_LB_Batt2_CellVoltage02_Msg)
  C_LB_Batt1_CellVoltage01_Msg/1 -> LiBa_Box1/1(C_LB_Batt1_CellVoltage01_Msg)
  C_LB_Batt2_Status03_Msg/1 -> LiBa_Box2/13(C_LB_Batt2_Status03_Msg)
  C_LB_Batt3_Status03_Timeout/1 -> LiBa_Box3/14(C_LB_Batt3_Status03_Timeout)
  C_LB_Batt2_Status01_Timeout/1 -> LiBa_Box2/10(C_LB_Batt2_Status01_Timeout)
  C_LB_Batt2_CellTemperature_Msg/1 -> LiBa_Box2/5(C_LB_Batt2_CellTemperature_Msg)
  C_LB_Batt2_Status01_Msg/1 -> LiBa_Box2/9(C_LB_Batt2_Status01_Msg)
  C_LB_Batt2_Status02_Msg/1 -> LiBa_Box2/11(C_LB_Batt2_Status02_Msg)
  C_LB_Batt2_InsulationMonitor_Timeout/1 -> LiBa_Box2/8(C_LB_Batt2_InsulationMonitor_Timeout)
  C_LB_Batt1_Status03_Timeout/1 -> LiBa_Box1/14(C_LB_Batt1_Status03_Timeout)
  C_LB_Batt1_Status02_Timeout/1 -> LiBa_Box1/12(C_LB_Batt1_Status02_Timeout)
  C_LB_Batt3_CellVoltage02_Timeout/1 -> LiBa_Box3/4(C_LB_Batt3_CellVoltage02_Timeout)
  LiBa_Box3/1(IP_LB_BattBox3_DataBus) -> Bus Creator/3
  C_LB_Batt1_Status01_Msg/1 -> LiBa_Box1/9(C_LB_Batt1_Status01_Msg)
  LiBa_Box2/1(IP_LB_BattBox2_DataBus) -> Bus Creator/2
  C_LB_Batt1_Status01_Timeout/1 -> LiBa_Box1/10(C_LB_Batt1_Status01_Timeout)
  C_LB_Batt1_CellTemperature_Msg/1 -> LiBa_Box1/5(C_LB_Batt1_CellTemperature_Msg)
  C_LB_Batt1_Status03_Msg/1 -> LiBa_Box1/13(C_LB_Batt1_Status03_Msg)
  C_LB_Batt1_CellVoltage02_Msg/1 -> LiBa_Box1/3(C_LB_Batt1_CellVoltage02_Msg)
  C_LB_Batt2_InsulationMonitor_Msg/1 -> LiBa_Box2/7(C_LB_Batt2_InsulationMonitor_Msg)
  C_LB_Batt3_CellTemperature_Timeout/1 -> LiBa_Box3/6(C_LB_Batt3_CellTemperature_Timeout)
  C_LB_Batt1_Status02_Msg/1 -> LiBa_Box1/11(C_LB_Batt1_Status02_Msg)
  C_LB_Batt1_InsulationMonitor_Msg/1 -> LiBa_Box1/7(C_LB_Batt1_InsulationMonitor_Msg)
  C_LB_Batt3_InsulationMonitor_Msg/1 -> LiBa_Box3/7(C_LB_Batt3_InsulationMonitor_Msg)
  C_LB_Batt1_CellVoltage02_Timeout/1 -> LiBa_Box1/4(C_LB_Batt1_CellVoltage02_Timeout)
  C_LB_Batt3_CellTemperature_Msg/1 -> LiBa_Box3/5(C_LB_Batt3_CellTemperature_Msg)
  C_LB_Batt1_CellTemperature_Timeout/1 -> LiBa_Box1/6(C_LB_Batt1_CellTemperature_Timeout)
  C_LB_Batt3_Status03_Msg/1 -> LiBa_Box3/13(C_LB_Batt3_Status03_Msg)
  C_LB_Batt3_CellVoltage01_Timeout/1 -> LiBa_Box3/2(C_LB_Batt3_CellVoltage01_Timeout)
  C_LB_Batt3_CellVoltage02_Msg/1 -> LiBa_Box3/3(C_LB_Batt3_CellVoltage02_Msg)
  C_LB_Batt3_Status01_Msg/1 -> LiBa_Box3/9(C_LB_Batt3_Status01_Msg)
  C_LB_Batt3_Status02_Msg/1 -> LiBa_Box3/11(C_LB_Batt3_Status02_Msg)
  C_LB_Batt3_Status01_Timeout/1 -> LiBa_Box3/10(C_LB_Batt3_Status01_Timeout)
  C_LB_Batt2_CellVoltage01_Msg/1 -> LiBa_Box2/1(C_LB_Batt2_CellVoltage01_Msg)
  C_LB_Batt2_CellTemperature_Timeout/1 -> LiBa_Box2/6(C_LB_Batt2_CellTemperature_Timeout)
  LiBa_Box1/1(IP_LB_BattBox1_DataBus) -> Bus Creator/1
  Bus Creator/1 -> IP_LB_BattBox_DataBus/1  "IP_LB_BattBox_DataBus"

== system ChiefMaster_TTC580/ChiefMaster/Input Processing/Subsystem2 ==
  C_UDC_Msg1 : Inport
  C_UDC_Msg1_Timeout : Inport  Port=2
  Bus Creator4 : BusCreator  Inputs=2
  Demux : Demux  Outputs=8
  NOT : Logic  Priority=5520  Operator=NOT  AllPortsSameDT=off  OutDataTypeStr=boolean
  Subsystem1 : Subsystem
  Subsystem3 : Subsystem
  Terminator{,1..4} (5 alike) : Terminator
  UDC_Databus : Outport
  wires:
  Demux/1 -> Subsystem1/1(byte1)
  Demux/3 -> Subsystem3/2(byte3)
  Demux/5 -> Terminator3/1
  Demux/7 -> Terminator1/1
  Demux/8 -> Terminator/1
  NOT/1 -> Subsystem1/Enable
  Demux/6 -> Terminator2/1
  Demux/4 -> Terminator4/1
  C_UDC_Msg1_Timeout/1 -> Subsystem3/3(C_TTC_Msg1_Timeout), NOT/1
  Subsystem3/1(IP_sLoadVoltage_Databus) -> Bus Creator4/2  "IP_sLoadVoltage_Databus"
  Demux/2 -> Subsystem3/1(byte2)
  Subsystem1/1(TTC_Status_Databus) -> Bus Creator4/1  "IP_UDC_Status_Databus"
  C_UDC_Msg1/1 -> Demux/1
  Bus Creator4/1 -> UDC_Databus/1  "UDC_Databus"

== system ChiefMaster_TTC580/ChiefMaster/Input Translation/Battery Selection ==
  IP_Databus : Inport
  Bus Creator1 : BusCreator  Inputs=3
  Bus Selector : BusSelector  OutputSignals=IP_Actia_BatBox_DataBus.IP_Actia_Batt1_Databus.IP_sActia_Batt1_Availability,IP_LB_BattBox_DataBus.IP_LB_BattBox1_DataBus.IP_boLiBa_Batt1_Availability,IP_Actia_BatBox_DataBus.IP_Actia_Batt2_Databus.IP_sActia_Batt2_Availability,IP_LB_BattBox_DataBus.IP_LB_BattBox2_DataBus.IP_boLiBa_Batt2_Availability,IP_Actia_BatBox_DataBus.IP_Actia_Batt3_Databus.IP_sActia_Batt3_Availability,IP_LB_BattBox_DataBus.IP_LB_BattBox3_DataBus.IP_boLiBa_Batt3_Availability
  ChartBatt1 : Stateflow chart  TreatAsAtomicUnit=on
      settings: RTWSystemCode=Reusable function  RTWFcnNameOpts=Use subsystem name  RTWFileNameOpts=Use subsystem name  PortSchema="{\"entries\":[{\"content\":{\"sides\":[{\"content\":{\"connectorIds\":[\"In2\",\"In1\"]},\"type\":\"ConnectorPlacement.EquallySpacedRectSide\",\"uuid\":\"2b0701cf-0d3a-4e22-94a9-5b959565742f\"},{\"content\":{\"connectorIds\":[\"Out1\"],\"side\":\"RIGHT\"},\"type\":\"ConnectorPlacement.EquallySpacedRectSide\",\"uuid\":\"37104f02-6f10-4442-ab75-d0614cbec1a3\"},{\"content\":{\"connectorIds\":[],\"side\":\"TOP\"},\"type\":\"ConnectorPlacement.EquallySpacedRectSide\",\"uuid\":\"8b67c104-2f49-4e69-88ba-a69e851b4ed9\"}]},\"type\":\"ConnectorPlacement.EquallySpacedConnector\",\"uuid\":\"8b838a0d-1f00-4c78-b54d-dbb2d1b41054\"}],\"packageUris\":[\"http://schema.mathworks.com/mf0/Connector/R2020b\"],\"version\":\"1.0\"}"
  ChartBatt3 : Stateflow chart  TreatAsAtomicUnit=on
      settings: RTWSystemCode=Reusable function  RTWFcnNameOpts=Use subsystem name  RTWFileNameOpts=Use subsystem name  PortSchema="{\"entries\":[{\"content\":{\"sides\":[{\"content\":{\"connectorIds\":[\"In2\",\"In1\"]},\"type\":\"ConnectorPlacement.EquallySpacedRectSide\",\"uuid\":\"2b0701cf-0d3a-4e22-94a9-5b959565742f\"},{\"content\":{\"connectorIds\":[\"Out1\"],\"side\":\"RIGHT\"},\"type\":\"ConnectorPlacement.EquallySpacedRectSide\",\"uuid\":\"37104f02-6f10-4442-ab75-d0614cbec1a3\"},{\"content\":{\"connectorIds\":[],\"side\":\"TOP\"},\"type\":\"ConnectorPlacement.EquallySpacedRectSide\",\"uuid\":\"8b67c104-2f49-4e69-88ba-a69e851b4ed9\"}]},\"type\":\"ConnectorPlacement.EquallySpacedConnector\",\"uuid\":\"8b838a0d-1f00-4c78-b54d-dbb2d1b41054\"}],\"packageUris\":[\"http://schema.mathworks.com/mf0/Connector/R2020b\"],\"version\":\"1.0\"}"
  Chartbatt2 : Stateflow chart  TreatAsAtomicUnit=on
      settings: RTWSystemCode=Reusable function  RTWFcnNameOpts=Use subsystem name  RTWFileNameOpts=Use subsystem name  PortSchema="{\"entries\":[{\"content\":{\"sides\":[{\"content\":{\"connectorIds\":[\"In2\",\"In1\"]},\"type\":\"ConnectorPlacement.EquallySpacedRectSide\",\"uuid\":\"2b0701cf-0d3a-4e22-94a9-5b959565742f\"},{\"content\":{\"connectorIds\":[\"Out1\"],\"side\":\"RIGHT\"},\"type\":\"ConnectorPlacement.EquallySpacedRectSide\",\"uuid\":\"37104f02-6f10-4442-ab75-d0614cbec1a3\"},{\"content\":{\"connectorIds\":[],\"side\":\"TOP\"},\"type\":\"ConnectorPlacement.EquallySpacedRectSide\",\"uuid\":\"8b67c104-2f49-4e69-88ba-a69e851b4ed9\"}]},\"type\":\"ConnectorPlacement.EquallySpacedConnector\",\"uuid\":\"8b838a0d-1f00-4c78-b54d-dbb2d1b41054\"}],\"packageUris\":[\"http://schema.mathworks.com/mf0/Connector/R2020b\"],\"version\":\"1.0\"}"
  Constant{1,3,5..6,9,11} (6 alike) : Constant  OutDataTypeStr=boolean
  Constant{2,4,7..8,10,12} (6 alike) : Constant  Value=0  OutDataTypeStr=boolean
  Switch{,1..5} (6 alike) : Switch  Criteria=u2 > Threshold  SaturateOnIntegerOverflow=off  InputSameDT=off
  IT_SelectBattery_Databus : Outport
  tag scope: Select_Battery1=global, Select_Battery2=global, Select_Battery3=global
  wires:
  Chartbatt2/1(BattSelect) -> Bus Creator1/2, [Select_Battery2]  "IT_u8Select_Battery2"
  Switch5/1 -> ChartBatt3/1(BattAvailable_LiBa)  "IP_boBatt3_LiBa_Availability"
  ChartBatt3/1(BattSelect) -> [Select_Battery3], Bus Creator1/3  "IT_u8Select_Battery3"
  Constant9/1 -> Switch4/1
  Switch1/1 -> ChartBatt1/1(BattAvailable_LiBa)  "IP_boBatt1_LiBa_Availability"
  Constant11/1 -> Switch5/1
  ChartBatt1/1(BattSelect) -> [Select_Battery1], Bus Creator1/1  "IT_u8Select_Battery1"
  Switch4/1 -> ChartBatt3/2(BattAvailable_Actia)  "IP_boBatt3_Actia_Availability"
  Constant10/1 -> Switch4/3
  Constant5/1 -> Switch3/1
  Switch2/1 -> Chartbatt2/2(BattAvailable_Actia)  "IP_boBatt2_Actia_Availability"
  Constant12/1 -> Switch5/3
  Constant8/1 -> Switch3/3
  Switch3/1 -> Chartbatt2/1(BattAvailable_LiBa)  "IP_boBatt2_LiBa_Availability"
  Constant4/1 -> Switch/3
  Constant2/1 -> Switch2/3
  Bus Selector/5 -> Switch4/2  "<IP_sActia_Batt3_Availability>"
  Constant7/1 -> Switch1/3
  Constant3/1 -> Switch/1
  Constant1/1 -> Switch2/1
  Bus Selector/4 -> Switch3/2  "<IP_boLiBa_Batt2_Availability>"
  Constant6/1 -> Switch1/1
  Switch/1 -> ChartBatt1/2(BattAvailable_Actia)  "IP_boBatt1_Actia_Availability"
  Bus Selector/6 -> Switch5/2  "<IP_boLiBa_Batt3_Availability>"
  Bus Selector/2 -> Switch1/2  "<IP_boLiBa_Batt1_Availability>"
  Bus Selector/3 -> Switch2/2  "<IP_sActia_Batt2_Availability>"
  Bus Creator1/1 -> IT_SelectBattery_Databus/1  "IT_SelectBattery_Databus"
  IP_Databus/1 -> Bus Selector/1
  Bus Selector/1 -> Switch/2  "<IP_sActia_Batt1_Availability>"

== system ChiefMaster_TTC580/ChiefMaster/Input Translation/Battery Signals ==
  IP_Databus : Inport
  IMD_Req_Databus : Inport  Port=2
  BatteryPackSignals : Subsystem  TreatAsAtomicUnit=on
  Bus Selector26 : BusSelector  OutputSignals=IP_Actia_BatBox_DataBus.IP_Actia_Batt1_Databus.IP_sActia_Batt1_VoltageAtSensor_V_Databus,IP_Actia_BatBox_DataBus.IP_Actia_Batt2_Databus.IP_sActia_Batt2_VoltageAtSensor_V_Databus,IP_Actia_BatBox_DataBus.IP_Actia_Batt3_Databus.IP_sActia_Batt3_VoltageAtSensor_V_Databus
  Bus Selector27 : BusSelector  OutputSignals=sData
  Bus Selector28 : BusSelector  OutputSignals=sData
  Bus Selector29 : BusSelector  OutputSignals=sData
  Bus Selector5 : BusSelector  OutputSignals=IP_Actia_BatBox_DataBus.IP_Actia_Batt1_Databus.IP_Actia_Batt1_MyStatus1_Databus.IP_boBatt1_ERROR_activ,IP_Actia_BatBox_DataBus.IP_Actia_Batt2_Databus.IP_Actia_Batt2_MyStatus1_Databus.IP_boBatt2_ERROR_activ,IP_Actia_BatBox_DataBus.IP_Actia_Batt3_Databus.IP_Actia_Batt3_MyStatus1_Databus.IP_boBatt3_ERROR_activ,IP_Actia_BatBox_DataBus.IP_Actia_Batt1_Databus.IP_Actia_Batt1_MyStatus1_Databus.IP_boBatt1_WARNING_activ,IP_Actia_BatBox_DataBus.IP_Actia_Batt2_Databus.IP_Actia_Batt2_MyStatus1_Databus.IP_boBatt2_WARNING_activ,IP_Actia_BatBox_DataBus.IP_Actia_Batt3_Databus.IP_Actia_Batt3_MyStatus1_Databus.IP_boBatt3_WARNING_activ
  Subsystem : Subsystem
  Subsystem1 : Subsystem
  Subsystem10 : Subsystem
  Subsystem11 : Subsystem
  Subsystem12 : Subsystem
  Subsystem14 : Subsystem
  Subsystem15 : Subsystem
  Subsystem2 : Subsystem
  Subsystem3 : Subsystem
  Subsystem4 : Subsystem
  Subsystem5 : Subsystem
  Subsystem6 : Subsystem
  Subsystem7 : Subsystem
  Subsystem8 : Subsystem
  Subsystem9 : Subsystem
  Terminator : Terminator
  Terminator1 : Terminator
  Terminator2 : Terminator
  IT_BatterySignal_Databus : Outport
  wires:
  Subsystem1/2(IP_boBMS_SDError_BB2) -> BatteryPackSignals/5(IP_boBMS_SDError_BB2)
  Subsystem/3(IP_sBMS_VtgInt_BB3) -> BatteryPackSignals/3(IP_sBMS_VtgInt_BB3)
  Subsystem1/1(IP_boBMS_SDError_BB1) -> BatteryPackSignals/4(IP_boBMS_SDError_BB1)
  IP_Databus/1 -> Subsystem15/1(IP_Databus), Subsystem8/1(IP_Databus), Bus Selector26/1, Subsystem10/1(IP_Databus), Subsystem14/1(IP_Databus), Subsystem7/1(IP_Databus), Subsystem11/1(IP_Databus), Subsystem9/1(IP_Databus), Subsystem12/1(IP_Databus), Subsystem4/1(IP_DataBus), Subsystem5/1(IP_DataBus), Subsystem3/1(IP_Databus), Subsystem6/1(IP_Databus), Bus Selector5/1, Subsystem2/1(IP_Databus), Subsystem1/1(IP_Databus), Subsystem/1(IP_Databus)
  Subsystem/1(IP_sBMS_VtgInt_BB1) -> BatteryPackSignals/1(IP_sBMS_VtgInt_BB1)
  Subsystem6/3(IP_sBMS_Current_BB3) -> BatteryPackSignals/18(IP_sBMS_Current_BB3)
  Subsystem10/1(IP_boBMS_IMD_Active_BB1) -> BatteryPackSignals/52(IP_boBMS_IMD_Active_BB1)
  Subsystem2/3(IP_boBMS_HV_REL_ON_BB3) -> BatteryPackSignals/9(IP_boBMS_HV_REL_ON_BB3)
  Subsystem3/3(IP_sBMS_SOC_BB3) -> BatteryPackSignals/21(IP_u8BMS_SOC_BB3)
  Bus Selector5/3 -> BatteryPackSignals/12(IP_boBMS_Error_BB3)  "<IP_boBatt3_ERROR_activ>"
  Subsystem9/3(IP_boBMS_HV_Minus_Sense_BB2) -> BatteryPackSignals/39(IP_boBMS_HV_Minus_Sense_BB2)
  Subsystem6/1(IP_sBMS_Current_BB1) -> BatteryPackSignals/16(IP_sBMS_Current_BB1)
  BatteryPackSignals/1(IT_BatterySignal_Databus) -> IT_BatterySignal_Databus/1
  Subsystem2/1(IP_boBMS_HV_REL_ON_BB1) -> BatteryPackSignals/7(IP_boBMS_HV_REL_ON_BB1)
  Bus Selector29/1 -> BatteryPackSignals/57(IP_sBMS_VtgExt_BB3_Sensor)  "<sData>"
  Subsystem8/2(IP_boBMS_Batt2_Availability) -> BatteryPackSignals/59(IP_boBMS_Batt2_Availability)
  Subsystem9/2(IP_boBMS_HV_Plus_Sense_BB1) -> BatteryPackSignals/38(IP_boBMS_HV_Plus_Sense_BB1)
  Subsystem7/3(IP_boBMS_InsulationReadyOK_B3) -> BatteryPackSignals/45(IP_boBMS_InsulationReadyOK_B3)
  Subsystem7/1(IP_boBMS_InsulationReadyOK_B1) -> BatteryPackSignals/43(IP_boBMS_InsulationReadyOK_B1)
  Subsystem11/1(IP_sBMS_InternalResistance_BB1) -> BatteryPackSignals/34(IP_sBMS_InternalResistance_BB1)
  Subsystem8/1(IP_boBMS_Batt1_Availability) -> BatteryPackSignals/58(IP_boBMS_Batt1_Availability)
  Subsystem9/6(IP_boBMS_HV_Plus_Sense_BB3) -> BatteryPackSignals/42(IP_boBMS_HV_Plus_Sense_BB3)
  Subsystem2/2(IP_boBMS_HV_REL_ON_BB2) -> BatteryPackSignals/8(IP_boBMS_HV_REL_ON_BB2)
  Subsystem/2(IP_sBMS_VtgInt_BB2) -> BatteryPackSignals/2(IP_sBMS_VtgInt_BB2)
  Subsystem9/1(IP_boBMS_HV_Minus_Sense_BB1) -> BatteryPackSignals/37(IP_boBMS_HV_Minus_Sense_BB1)
  Subsystem6/2(IP_sBMS_Current_BB2) -> BatteryPackSignals/17(IP_sBMS_Current_BB2)
  Subsystem11/2(IP_sBMS_InternalResistance_BB2) -> BatteryPackSignals/35(IP_sBMS_InternalResistance_BB2)
  Subsystem9/4(IP_boBMS_HV_Plus_Sense_BB2) -> BatteryPackSignals/40(IP_boBMS_HV_Plus_Sense_BB2)
  Bus Selector26/3 -> Bus Selector29/1  "<IP_sActia_Batt3_VoltageAtSensor_V_Databus>"
  Subsystem7/2(IP_boBMS_InsulationReadyOK_B2) -> BatteryPackSignals/44(IP_boBMS_InsulationReadyOK_B2)
  Subsystem10/3(IP_boBMS_IMD_Active_BB3) -> BatteryPackSignals/54(IP_boBMS_IMD_Active_BB3)
  Subsystem1/3(IP_boBMS_SDError_BB3) -> BatteryPackSignals/6(IP_boBMS_SDError_BB3)
  Bus Selector26/1 -> Bus Selector27/1  "<IP_sActia_Batt1_VoltageAtSensor_V_Databus>"
  Subsystem3/1(IP_sBMS_SOC_BB1) -> BatteryPackSignals/19(IP_u8BMS_SOC_BB1)
  Subsystem4/2(IP_sBMS_DisChargeCurrentPrognosis_BB2) -> BatteryPackSignals/26(IP_sBMS_DisChargeCurrentPrognosis_BB2)
  Subsystem4/3(IP_sBMS_DisChargeCurrentPrognosis_BB3) -> BatteryPackSignals/27(IP_sBMS_DisChargeCurrentPrognosis_BB3)
  Bus Selector5/4 -> BatteryPackSignals/13(IP_boBMS_Warning_BB1)  "<IP_boBatt1_WARNING_activ>"
  Subsystem5/2(IP_sBMS_ChargeCurrentPrognosis_BB2) -> BatteryPackSignals/23(IP_sBMS_ChargeCurrentPrognosis_BB2)
  Subsystem9/5(IP_boBMS_HV_Minus_Sense_BB3) -> BatteryPackSignals/41(IP_boBMS_HV_Minus_Sense_BB3)
  Bus Selector26/2 -> Bus Selector28/1  "<IP_sActia_Batt2_VoltageAtSensor_V_Databus>"
  Subsystem11/3(IP_sBMS_InternalResistance_BB3) -> BatteryPackSignals/36(IP_sBMS_InternalResistance_BB3)
  Bus Selector5/1 -> BatteryPackSignals/10(IP_boBMS_Error_BB1)  "<IP_boBatt1_ERROR_activ>"
  Bus Selector5/5 -> BatteryPackSignals/14(IP_boBMS_Warning_BB2)  "<IP_boBatt2_WARNING_activ>"
  Subsystem4/1(IP_sBMS_DisChargeCurrentPrognosis_BB1) -> BatteryPackSignals/25(IP_sBMS_DisChargeCurrentPrognosis_BB1)
  Subsystem3/2(IP_sBMS_SOC_BB2) -> BatteryPackSignals/20(IP_u8BMS_SOC_BB2)
  IMD_Req_Databus/1 -> Subsystem7/2(IMD_Req_Databus), Subsystem10/2(IMD_Req_Databus)
  Bus Selector27/1 -> BatteryPackSignals/55(IP_sBMS_VtgExt_BB1_Sensor)  "<sData>"
  Subsystem10/2(IP_boBMS_IMD_Active_BB2) -> BatteryPackSignals/53(IP_boBMS_IMD_Active_BB2)
  Subsystem5/3(IP_sBMS_ChargeCurrentPrognosis_BB3) -> BatteryPackSignals/24(IP_sBMS_ChargeCurrentPrognosis_BB3)
  Bus Selector5/6 -> BatteryPackSignals/15(IP_boBMS_Warning_BB3)  "<IP_boBatt3_WARNING_activ>"
  Bus Selector28/1 -> BatteryPackSignals/56(IP_sBMS_VtgExt_BB2_Sensor)  "<sData>"
  Bus Selector5/2 -> BatteryPackSignals/11(IP_boBMS_Error_BB2)  "<IP_boBatt2_ERROR_activ>"
  Subsystem5/1(IP_sBMS_ChargeCurrentPrognosis_BB1) -> BatteryPackSignals/22(IP_sBMS_ChargeCurrentPrognosis_BB1)
  Subsystem8/3(IP_boBMS_Batt3_Availability) -> BatteryPackSignals/60(IP_boBMS_Batt3_Availability)
  Subsystem12/1(IP_boBMS_InsulationResistance_kOhm_BB1) -> BatteryPackSignals/28(IP_sBMS_InsulationResistance_BB1)
  Subsystem12/2(IP_boBMS_InsulationResistance_kOhm_BB2) -> BatteryPackSignals/29(IP_sBMS_InsulationResistance_BB2)
  Subsystem12/3(IP_boBMS_InsulationResistance_kOhm_BB3) -> BatteryPackSignals/30(IP_sBMS_InsulationResistance_BB3)
  Subsystem12/4(IP_boBMS_InsulationResistance_Minus_kOhm_BB1) -> BatteryPackSignals/31(IP_boBMS_InsulationResistance_Minus_kOhm_BB1)
  Subsystem12/5(IP_boBMS_InsulationResistance_Minus_kOhm_BB2) -> BatteryPackSignals/32(IP_boBMS_InsulationResistance_Minus_kOhm_BB2)
  Subsystem12/6(IP_boBMS_InsulationResistance_Minus_kOhm_BB3) -> BatteryPackSignals/33(IP_boBMS_InsulationResistance_Minus_kOhm_BB3)
  Subsystem14/1(IP_sBMS_MinCellVoltage_BB1) -> BatteryPackSignals/46(IP_sBMS_MinCellVoltage_BB1)
  Subsystem14/2(IP_sBMS_MinCellVoltage_BB2) -> BatteryPackSignals/47(IP_sBMS_MinCellVoltage_BB2)
  Subsystem14/3(IP_sBMS_MinCellVoltage_BB3) -> BatteryPackSignals/48(IP_sBMS_MinCellVoltage_BB3)
  Subsystem14/4(IP_sBMS_MaxCellVoltage_BB1) -> BatteryPackSignals/49(IP_sBMS_MaxCellVoltage_BB1)
  Subsystem14/5(IP_sBMS_MaxCellVoltage_BB2) -> BatteryPackSignals/50(IP_sBMS_MaxCellVoltage_BB2)
  Subsystem14/6(IP_sBMS_MaxCellVoltage_BB3) -> BatteryPackSignals/51(IP_sBMS_MaxCellVoltage_BB3)
  Subsystem15/1(IP_sBMS_MinTemp_degC_BB1) -> BatteryPackSignals/61(IP_sBMS_MinTemp_degC_BB1)
  Subsystem15/2(IP_sBMS_MaxTemp_degC_BB1) -> BatteryPackSignals/62(IP_sBMS_MaxTemp_degC_BB1)
  Subsystem15/3(IP_sBMS_MinTemp_degC_BB2) -> BatteryPackSignals/63(IP_sBMS_MinTemp_degC_BB2)
  Subsystem15/4(IP_sBMS_MaxTemp_degC_BB2) -> BatteryPackSignals/64(IP_sBMS_MaxTemp_degC_BB2)
  Subsystem15/5(IP_sBMS_MinTemp_degC_BB3) -> BatteryPackSignals/65(IP_sBMS_MinTemp_degC_BB3)
  Subsystem15/6(IP_sBMS_MaxTemp_degC_BB3) -> BatteryPackSignals/66(IP_sBMS_MaxTemp_degC_BB3)
  Subsystem12/7(IP_LiBa_Insulation_OK_BB1) -> Terminator/1
  Subsystem12/8(IP_LiBa_Insulation_OK_BB2) -> Terminator1/1
  Subsystem12/9(IP_LiBa_Insulation_OK_BB3) -> Terminator2/1
